simulink model "fuzzy49_fuzzy9sim"  (R2019a)
settings: Solver=VariableStepAuto  StartTime=0.0  StopTime=10  RelTol=1e-3
settings Model: Creator=ancem  LastModifiedBy=ancem

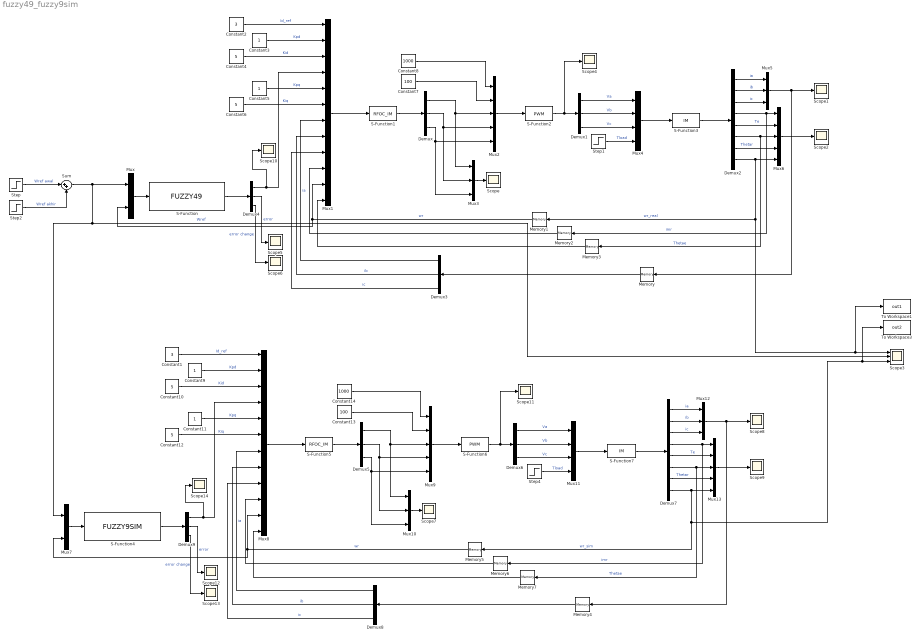
== system fuzzy49_fuzzy9sim ==
  Constant1 : Constant  Value=3
  Constant{4,6,10,12} (4 alike) : Constant  Value=5
  Constant{3,5,9,11} (4 alike) : Constant
  Constant13 : Constant  Value=100
  Constant14 : Constant  Value=1000
  Constant2 : Constant  Value=3
  Constant7 : Constant  Value=100
  Constant8 : Constant  Value=1000
  Demux{,1,3..6,8..9} (8 alike) : Demux  Outputs=3
  Demux2 : Demux  Outputs=8
  Demux7 : Demux  Outputs=8
  Memory{,1..7} (8 alike) : Memory
  Mux : Mux  Inputs=2
  Mux1 : Mux  Inputs=12
  Mux{3,5,10,12} (4 alike) : Mux  Inputs=3
  Mux11 : Mux
  Mux{2,6,9,13} (4 alike) : Mux  Inputs=5
  Mux4 : Mux
  Mux7 : Mux  Inputs=2
  Mux8 : Mux  Inputs=12
  S-Function : S-Function  FunctionName=FUZZY49  SFunctionDeploymentMode=off  EnableBusSupport=off
  S-Function1 : S-Function  FunctionName=RFOC_IM  SFunctionDeploymentMode=off  EnableBusSupport=off
  S-Function2 : S-Function  FunctionName=PWM  SFunctionDeploymentMode=off  EnableBusSupport=off
  S-Function3 : S-Function  FunctionName=IM  SFunctionDeploymentMode=off  EnableBusSupport=off
  S-Function4 : S-Function  FunctionName=FUZZY9SIM  SFunctionDeploymentMode=off  EnableBusSupport=off
  S-Function5 : S-Function  FunctionName=RFOC_IM  SFunctionDeploymentMode=off  EnableBusSupport=off
  S-Function6 : S-Function  FunctionName=PWM  SFunctionDeploymentMode=off  EnableBusSupport=off
  S-Function7 : S-Function  FunctionName=IM  SFunctionDeploymentMode=off  EnableBusSupport=off
  Scope{,1..2,4..14} (14 alike) : Scope
  Scope3 : Scope  NumInputPorts=3
  Step : Step  After=10  SampleTime=0
  Step1 : Step  Time=3  After=0  SampleTime=0
  Step2 : Step  Time=5  After=-20  SampleTime=0
  Step4 : Step  Time=3  After=0  SampleTime=0
  Sum : Sum  Inputs=|++
  To Workspace1 : ToWorkspace  VariableName=out1  SampleTime=-1
  To Workspace3 : ToWorkspace  VariableName=out2  SampleTime=-1
  wires:
  Demux3/1 -> Mux1/7  "ia"
  Demux1/2 -> Mux4/2  "Vb"
  Demux2/4 -> Memory2/1, Mux6/1  "imr"
  Mux/1 -> S-Function/1
  Demux3/2 -> Mux1/8  "ib"
  Memory1/1 -> Mux/2, Mux1/11  "wr"
  Demux1/3 -> Mux4/3  "Vc"
  Memory2/1 -> Mux1/10
  Demux/2 -> Mux3/2, Mux2/4
  Demux2/5 -> Mux6/2  "Te"
  S-Function3/1 -> Demux2/1
  Mux3/1 -> Scope/1
  Demux/1 -> Mux2/3, Mux3/1
  Constant2/1 -> Mux1/1  "Id_ref"
  Mux5/1 -> Memory/1, Scope1/1
  Demux2/6 -> Mux6/3, Memory3/1  "Thetae"
  Demux2/3 -> Mux5/3  "ic"
  Constant5/1 -> Mux1/5  "Kpq"
  S-Function2/1 -> Scope4/1, Demux1/1
  Demux2/2 -> Mux5/2  "ib"
  Constant8/1 -> Mux2/1
  Memory3/1 -> Mux1/12
  Step1/1 -> Mux4/4  "Tload"
  Demux2/1 -> Mux5/1  "ia"
  Demux1/1 -> Mux4/1  "Va"
  Mux2/1 -> S-Function2/1
  Demux/3 -> Mux3/3, Mux2/5
  Mux1/1 -> S-Function1/1
  S-Function1/1 -> Demux/1
  Constant6/1 -> Mux1/6  "Kiq"
  Constant4/1 -> Mux1/3  "Kid"
  Mux6/1 -> Scope2/1
  Memory/1 -> Demux3/1
  Constant3/1 -> Mux1/2  "Kpd"
  Constant7/1 -> Mux2/2
  Demux3/3 -> Mux1/9  "ic"
  Demux2/7 -> Mux6/4  "Thetar"
  Mux4/1 -> S-Function3/1
  S-Function/1 -> Demux4/1
  Demux4/1 -> Scope10/1, Mux1/4
  Demux4/2 -> Scope5/1  "error"
  Demux4/3 -> Scope6/1  "error change"
  Step/1 -> Sum/1  "Wref awal"
  Sum/1 -> Mux/1, Mux7/1, Scope3/2  "Wref"
  Step2/1 -> Sum/2  "Wref akhir"
  Constant12/1 -> Mux8/6  "Kiq"
  Mux10/1 -> Scope7/1
  Demux5/3 -> Mux10/3, Mux9/5
  Constant14/1 -> Mux9/1
  Demux7/6 -> Mux13/3, Memory7/1  "Thetae"
  Memory5/1 -> Mux7/2, Mux8/11  "wr"
  Demux8/2 -> Mux8/8  "ib"
  Demux6/1 -> Mux11/1  "Va"
  Mux13/1 -> Scope9/1
  S-Function6/1 -> Scope11/1, Demux6/1
  Mux8/1 -> S-Function5/1
  Step4/1 -> Mux11/4  "Tload"
  Demux8/1 -> Mux8/7  "ia"
  Memory7/1 -> Mux8/12
  Demux7/4 -> Memory6/1, Mux13/1  "imr"
  Mux11/1 -> S-Function7/1
  Mux7/1 -> S-Function4/1
  Mux12/1 -> Memory4/1, Scope8/1
  Mux9/1 -> S-Function6/1
  Demux7/7 -> Mux13/4  "Thetar"
  Constant9/1 -> Mux8/2  "Kpd"
  Demux7/2 -> Mux12/2  "ib"
  Constant13/1 -> Mux9/2
  Constant10/1 -> Mux8/3  "Kid"
  Demux5/1 -> Mux9/3, Mux10/1
  Constant1/1 -> Mux8/1  "Id_ref"
  S-Function4/1 -> Demux9/1
  Demux9/3 -> Scope13/1  "error change"
  S-Function7/1 -> Demux7/1
  Demux6/2 -> Mux11/2  "Vb"
  Demux7/5 -> Mux13/2  "Te"
  Demux9/2 -> Scope12/1  "error"
  S-Function5/1 -> Demux5/1
  Memory4/1 -> Demux8/1
  Demux7/1 -> Mux12/1  "ia"
  Constant11/1 -> Mux8/5  "Kpq"
  Demux9/1 -> Scope14/1, Mux8/4
  Demux6/3 -> Mux11/3  "Vc"
  Demux8/3 -> Mux8/9  "ic"
  Demux7/3 -> Mux12/3  "ic"
  Demux5/2 -> Mux10/2, Mux9/4
  Memory6/1 -> Mux8/10
  Demux7/8 -> Mux13/5, To Workspace3/1, Scope3/3, Memory5/1  "wr_sim"
  Demux2/8 -> Mux6/5, To Workspace1/1, Scope3/1, Memory1/1  "wr_real"
